simulink model "Predictor_de_smith"  (R2014a)
settings: Solver=ode45  StartTime=0.0  StopTime=1000  RelTol=1e-3
values from neighbouring files (symbols this model uses):
  Fh0 = 0.8946    [Seccion_4.m]
libraries: simulink_need_slupdate x1
settings Model: Creator=lraff  LastModifiedBy=lraff

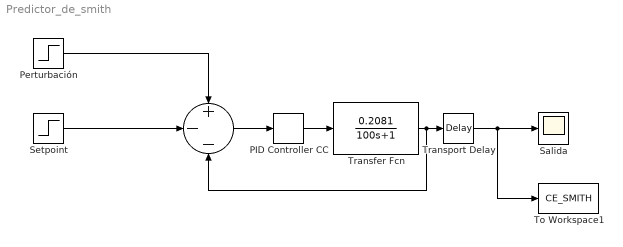
== system Predictor_de_smith ==
  " " : Sum  Inputs=+--
  PID Controller CC : simulink_need_slupdate/PID Controller  P=24.0269  I=0.240269  D=0
  Perturbación : Step  Time=100  Before=Fh0  After=Fh0*1.02  SampleTime=1
  "Salida " : Scope
  Setpoint : Step  Time=0  Before=Fh0  After=Fh0  SampleTime=1
  To Workspace1 : ToWorkspace  VariableName=CE_SMITH  SaveFormat=Structure With Time
  Transfer Fcn : TransferFcn  Numerator=[0.2081]  Denominator=[100 1]
  Transport Delay : TransportDelay  DelayTime=21.8
  wires:
  " "/1 -> PID Controller CC/1
  Transfer Fcn/1 -> " "/3, Transport Delay/1
  Transport Delay/1 -> To Workspace1/1, "Salida "/1
  Setpoint/1 -> " "/2
  PID Controller CC/1 -> Transfer Fcn/1
  Perturbación/1 -> " "/1
